simulink model "ClosedLoop_AdaptivePID_N256_B64"  (R2024a)
settings: Solver=VariableStepAuto  StartTime=0.0  StopTime=10.0  RelTol=1e-3
undefined symbols (not defined in the file): A, B, C, N, torch
libraries: pycoexlib x1
settings Model: Creator=mahariansyah  LastModifiedBy=mahariansyah

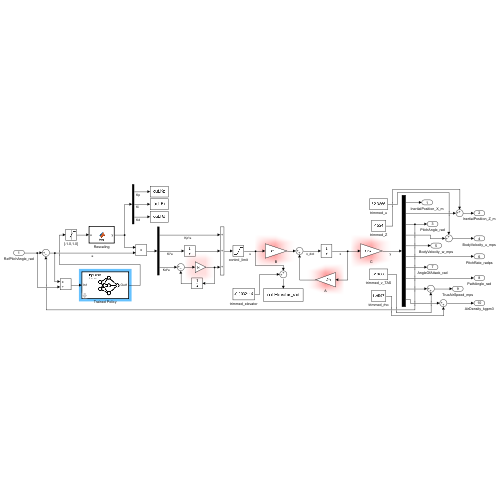
[thumbnail: Simulink's stored preview of the top-level diagram]
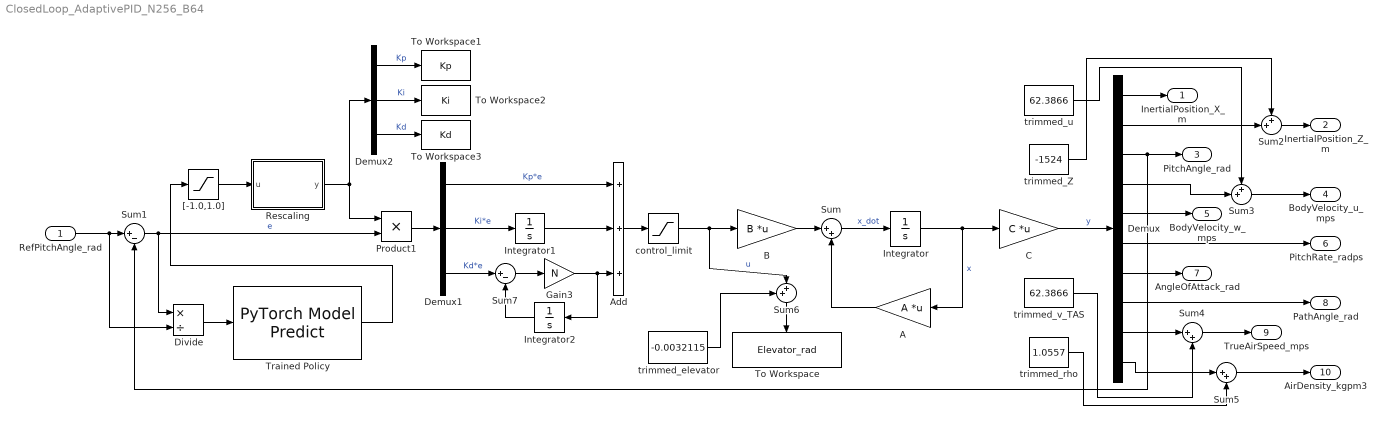
== system ClosedLoop_AdaptivePID_N256_B64 ==
  RefPitchAngle_rad : Inport
  A : Gain  Gain=A  Multiplication=Matrix(K*u)
  Add : Sum  Inputs=+++
  B : Gain  Gain=B  Multiplication=Matrix(K*u)
  C : Gain  Gain=C  Multiplication=Matrix(K*u)
  Demux : Demux  Outputs=10
  Demux1 : Demux  Outputs=3
  Demux2 : Demux  Outputs=3
  Divide : Product  Inputs=*/
  Gain3 : Gain  Gain=N
  Integrator : Integrator
  Integrator1 : Integrator
  Integrator2 : Integrator
  Product1 : Product
  Rescaling : MATLAB Function  TreatAsAtomicUnit=on
  Sum : Sum  Inputs=|++
  Sum1 : Sum  Inputs=|+-
  Sum2 : Sum  Inputs=++|
  Sum3 : Sum  Inputs=++|
  Sum4 : Sum  Inputs=|++
  Sum5 : Sum  Inputs=|++
  Sum6 : Sum  Inputs=++|
  Sum7 : Sum  Inputs=|+-
  To Workspace : ToWorkspace  VariableName=Elevator_rad  SaveFormat=Timeseries  SampleTime=-1
  To Workspace1 : ToWorkspace  VariableName=Kp  SaveFormat=Timeseries  SampleTime=-1
  To Workspace2 : ToWorkspace  VariableName=Ki  SaveFormat=Timeseries  SampleTime=-1
  To Workspace3 : ToWorkspace  VariableName=Kd  SaveFormat=Timeseries  SampleTime=-1
  Trained Policy : pycoexlib/PyTorch Model Predict  LoadCommandPopup=torch.load()  ModelFile=C:\Users\mahariansyah\OneDrive - HKUST Connect\Control_Project\6_Intelligent_method_rl_adaptive_pids\trained_models\pytorch_model_n256_b64.pt  InputTable={ 'In1', 'float32', '', 'inherit' }  OutputTable={ 'Out1', '', '' }  SampleTime=-1  TorchLoadCommand=torch.load()  InputDatatypes=float32  InputNumDims=inherit  InputPermutations=[]  OutputPermutations=[]  PythonCoexecutionBlockType=PyTorchModelBlock  VariableOutputMaxSizes=[]
  "[-1.0,1.0]" : Saturate  UpperLimit=1.0  LowerLimit=-1.0
  control_limit : Saturate  UpperLimit=30/180*pi  LowerLimit=-30/180*pi
  trimmed_Z : Constant  Value=-1524
  trimmed_elevator : Constant  Value=-0.0032115
  trimmed_rho : Constant  Value=1.0557
  trimmed_u : Constant  Value=62.3866
  trimmed_v_TAS : Constant  Value=62.3866
  InertialPosition_X_m : Outport
  InertialPosition_Z_m : Outport  Port=2
  PitchAngle_rad : Outport  Port=3
  BodyVelocity_u_mps : Outport  Port=4
  BodyVelocity_w_mps : Outport  Port=5
  PitchRate_radps : Outport  Port=6
  AngleOfAttack_rad : Outport  Port=7
  PathAngle_rad : Outport  Port=8
  TrueAirSpeed_mps : Outport  Port=9
  AirDensity_kgpm3 : Outport  Port=10
  wires:
  Integrator/1 -> A/1, C/1  "x"
  Sum/1 -> Integrator/1  "x_dot"
  A/1 -> Sum/2
  B/1 -> Sum/1
  Add/1 -> control_limit/1
  RefPitchAngle_rad/1 -> Divide/2, Sum1/1
  Sum1/1 -> Divide/1, Product1/2  "e"
  Demux/1 -> InertialPosition_X_m/1
  Demux/3 -> PitchAngle_rad/1, Sum1/2
  Demux/5 -> BodyVelocity_w_mps/1
  Demux/6 -> PitchRate_radps/1
  Demux/7 -> AngleOfAttack_rad/1
  Demux/8 -> PathAngle_rad/1
  Sum2/1 -> InertialPosition_Z_m/1
  Demux/2 -> Sum2/2
  trimmed_Z/1 -> Sum2/1
  Demux/4 -> Sum3/2
  Sum3/1 -> BodyVelocity_u_mps/1
  trimmed_u/1 -> Sum3/1
  Sum4/1 -> TrueAirSpeed_mps/1
  Demux/9 -> Sum4/1
  trimmed_v_TAS/1 -> Sum4/2
  Sum5/1 -> AirDensity_kgpm3/1
  Demux/10 -> Sum5/1
  trimmed_rho/1 -> Sum5/2
  C/1 -> Demux/1  "y"
  Integrator1/1 -> Add/2
  Demux1/2 -> Integrator1/1  "Ki*e"
  Gain3/1 -> Integrator2/1, Add/3
  Sum7/1 -> Gain3/1
  Integrator2/1 -> Sum7/2
  Sum6/1 -> To Workspace/1
  trimmed_elevator/1 -> Sum6/1
  control_limit/1 -> B/1, Sum6/2  "u"
  Divide/1 -> Trained Policy/1
  Trained Policy/1 -> "[-1.0,1.0]"/1
  "[-1.0,1.0]"/1 -> Rescaling/1(u)
  Rescaling/1(y) -> Demux2/1, Product1/1
  Product1/1 -> Demux1/1
  Demux1/3 -> Sum7/1  "Kd*e"
  Demux1/1 -> Add/1  "Kp*e"
  Demux2/1 -> To Workspace1/1  "Kp"
  Demux2/2 -> To Workspace2/1  "Ki"
  Demux2/3 -> To Workspace3/1  "Kd"

== matlab function ClosedLoop_AdaptivePID_N256_B64/Rescaling ==
  data: u input; y output
function y = fcn(u)
u1 = 1.5*(u(1)+1.0)-3.0;
u2 = 1.5*(u(2)+1.0)-3.0;
u3 = 1.5*(u(3)+1.0)-3.0;
y = [u1; u2; u3];
